simulink model "HANcoder_E407_TTA_Controller_v3"  (R2018b)
settings: Solver=FixedStepDiscrete  StartTime=0.0  StopTime=1  FixedStep=0.01  RelTol=1e-3
PreLoadFcn:
  | librarySetup
  | eval([bdroot,'_startup']) %Calling [modelName]_startup.m
values from neighbouring files (symbols this model uses):
  basic_cycle_duration_bc0 = TM_Reset_Board   + COMP_duration    (= 212)    [HANcoder_E407_TTA_Controller_v3_startup.m]
  basic_cycle_duration_bc1 = TM_Reset_Var_bc1 + COMP_duration    (= 288)    [HANcoder_E407_TTA_Controller_v3_startup.m]
  comm_delay_estimation1 = round(comm_delay_measured1*hardware_granularity/frequency_IRQ)    [HANcoder_E407_TTA_Controller_v3_startup.m]
  comm_delay_estimation2 = round(comm_delay_measured2*hardware_granularity/frequency_IRQ)    [HANcoder_E407_TTA_Controller_v3_startup.m]
  COMM_Period = 40    [HANcoder_E407_TTA_Controller_v3_startup.m]
  COMM_Phase1 = 5    [HANcoder_E407_TTA_Controller_v3_startup.m]
  COMM_Phase2 = 8    [HANcoder_E407_TTA_Controller_v3_startup.m]
  COMP_duration = 4    [HANcoder_E407_TTA_Controller_v3_startup.m]
  Controller1_Board = 1    [HANcoder_E407_TTA_Controller_v3_startup.m]
  Controller2_Board = 2    [HANcoder_E407_TTA_Controller_v3_startup.m]
  Controller3_Board = 3    [HANcoder_E407_TTA_Controller_v3_startup.m]
  delta_a_set = Simulink.Parameter    [HANcoder_E407_TTA_Controller_v3_startup.m]
  delta_f_set = Simulink.Parameter    [HANcoder_E407_TTA_Controller_v3_startup.m]
  delta_max = 1    [HANcoder_E407_TTA_Controller_v3_startup.m]
  delta_min = -1    [HANcoder_E407_TTA_Controller_v3_startup.m]
  delta_precision = 6    [HANcoder_E407_TTA_Controller_v3_startup.m]
  e_width = 0.1    [HANcoder_E407_TTA_Controller_v3_startup.m]
  frequency_IRQ = 100    [HANcoder_E407_TTA_Controller_v3_startup.m]
  HANtuneOverride = Simulink.Parameter    [HANcoder_E407_TTA_Controller_v3_startup.m]
  hardware_granularity = 1000000    [HANcoder_E407_TTA_Controller_v3_startup.m]
  I_a = 2.25    [HANcoder_E407_TTA_Controller_v3_startup.m]
  I_f = 2.25    [HANcoder_E407_TTA_Controller_v3_startup.m]
  idle_time_init = basic_cycle_duration_bc0 + basic_cycle_duration_bc1    (= 500)    [HANcoder_E407_TTA_Controller_v3_startup.m]
  Input_Gen_Board = 4    [HANcoder_E407_TTA_Controller_v3_startup.m]
  LA_Clock_Gr = 1    [HANcoder_E407_TTA_Controller_v3_startup.m]
  LA_COMM_Err = 0    [HANcoder_E407_TTA_Controller_v3_startup.m]
  LA_MEX_Flag = 0    [HANcoder_E407_TTA_Controller_v3_startup.m]
  LA_Task_Act = 1    [HANcoder_E407_TTA_Controller_v3_startup.m]
  m_v = 100.0    (= 100)    [HANcoder_E407_TTA_Controller_v3_startup.m]
  Master_Role = 1    [HANcoder_E407_TTA_Controller_v3_startup.m]
  matrix_cycle_duration = basic_cycle_duration_bc0 + basic_cycle_duration_bc1    (= 500)    [HANcoder_E407_TTA_Controller_v3_startup.m]
  matrix_rows = 2    [HANcoder_E407_TTA_Controller_v3_startup.m]
  max_num_msgs_CAN1 = 2^Tx_bit_number-1    (= 7)    [HANcoder_E407_TTA_Controller_v3_startup.m]
  max_num_msgs_CAN2 = max_num_msgs_CAN1    (= 7)    [HANcoder_E407_TTA_Controller_v3_startup.m]
  OutControl1_ID = 23    [HANcoder_E407_TTA_Controller_v3_startup.m]
  OutControl2_ID = 24    [HANcoder_E407_TTA_Controller_v3_startup.m]
  OutEmulator_ID = 25    [HANcoder_E407_TTA_Controller_v3_startup.m]
  R_al = 0.10    (= 0.1)    [HANcoder_E407_TTA_Controller_v3_startup.m]
  R_ar = 0.10    (= 0.1)    [HANcoder_E407_TTA_Controller_v3_startup.m]
  R_fl = 0.10    (= 0.1)    [HANcoder_E407_TTA_Controller_v3_startup.m]
  R_fr = 0.10    (= 0.1)    [HANcoder_E407_TTA_Controller_v3_startup.m]
  SensorValues_ID = 22    [HANcoder_E407_TTA_Controller_v3_startup.m]
  SetValues_ID = 21    [HANcoder_E407_TTA_Controller_v3_startup.m]
  Slave_Role = 2    [HANcoder_E407_TTA_Controller_v3_startup.m]
  speed_k_d = Simulink.Parameter    [HANcoder_E407_TTA_Controller_v3_startup.m]
  speed_k_i = Simulink.Parameter    [HANcoder_E407_TTA_Controller_v3_startup.m]
  speed_k_p = Simulink.Parameter    [HANcoder_E407_TTA_Controller_v3_startup.m]
  speed_max = 10    [HANcoder_E407_TTA_Controller_v3_startup.m]
  speed_min = -10    [HANcoder_E407_TTA_Controller_v3_startup.m]
  speed_precision = 3    [HANcoder_E407_TTA_Controller_v3_startup.m]
  Sync_ID = 1    [HANcoder_E407_TTA_Controller_v3_startup.m]
  tau_max = 5    [HANcoder_E407_TTA_Controller_v3_startup.m]
  tau_min = -5    [HANcoder_E407_TTA_Controller_v3_startup.m]
  tau_range = abs(tau_max) + abs(tau_min)    [HANcoder_E407_TTA_Controller_v3_startup.m]
  theta_max = 2    [HANcoder_E407_TTA_Controller_v3_startup.m]
  theta_min = -2    [HANcoder_E407_TTA_Controller_v3_startup.m]
  theta_precision = 5    [HANcoder_E407_TTA_Controller_v3_startup.m]
  Tl_a = 0.6    [HANcoder_E407_TTA_Controller_v3_startup.m]
  Tl_f = 0.6    [HANcoder_E407_TTA_Controller_v3_startup.m]
  TM_Check_Output_Control1 = TM_COMM_Output_Control1 + COMM_duration    (= 188)    [HANcoder_E407_TTA_Controller_v3_startup.m]
  TM_Check_Output_Control2 = TM_COMM_Output_Control2 + COMM_duration    (= 232)    [HANcoder_E407_TTA_Controller_v3_startup.m]
  TM_Check_Output_Emulator = TM_COMM_Output_Emulator + COMM_duration    (= 280)    [HANcoder_E407_TTA_Controller_v3_startup.m]
  TM_Check_Sensor_Values = TM_COMM_Sensor_Values + COMM_duration    (= 132)    [HANcoder_E407_TTA_Controller_v3_startup.m]
  TM_Check_Set_Values = TM_COMM_Set_Values + COMM_duration    (= 88)    [HANcoder_E407_TTA_Controller_v3_startup.m]
  TM_Check_Sync = TM_COMM_Sync   + COMM_duration    (= 40)    [HANcoder_E407_TTA_Controller_v3_startup.m]
  TM_Check_TOuts = TM_Count_Vote3 + COMP_duration    (= 196)    [HANcoder_E407_TTA_Controller_v3_startup.m]
  TM_Check_Vote1 = TM_COMM_Vote1  + COMM_duration    (= 92)    [HANcoder_E407_TTA_Controller_v3_startup.m]
  TM_Check_Vote2 = TM_COMM_Vote2  + COMM_duration    (= 140)    [HANcoder_E407_TTA_Controller_v3_startup.m]
  TM_Check_Vote3 = TM_COMM_Vote3  + COMM_duration    (= 188)    [HANcoder_E407_TTA_Controller_v3_startup.m]
  TM_COMM_Output_Control1 = TM_Velocity + COMP_duration    (= 148)    [HANcoder_E407_TTA_Controller_v3_startup.m]
  TM_COMM_Output_Control2 = TM_Check_Output_Control1 + COMP_duration    (= 192)    [HANcoder_E407_TTA_Controller_v3_startup.m]
  TM_COMM_Output_Emulator = TM_TMR + COMP_duration    (= 240)    [HANcoder_E407_TTA_Controller_v3_startup.m]
  TM_COMM_Sensor_Values = TM_Check_Set_Values + COMP_duration    (= 92)    [HANcoder_E407_TTA_Controller_v3_startup.m]
  TM_COMM_Set_Values = TM_Update_LT + COMP_duration    (= 48)    [HANcoder_E407_TTA_Controller_v3_startup.m]
  TM_COMM_Sync = basic_cycle_start    (= 0)    [HANcoder_E407_TTA_Controller_v3_startup.m]
  TM_COMM_Vote1 = TM_Vote_Dec    + COMP_duration    (= 52)    [HANcoder_E407_TTA_Controller_v3_startup.m]
  TM_COMM_Vote2 = TM_Count_Vote1 + COMP_duration    (= 100)    [HANcoder_E407_TTA_Controller_v3_startup.m]
  TM_COMM_Vote3 = TM_Count_Vote2 + COMP_duration    (= 148)    [HANcoder_E407_TTA_Controller_v3_startup.m]
  TM_Count_Vote1 = TM_Check_Vote1 + COMP_duration    (= 96)    [HANcoder_E407_TTA_Controller_v3_startup.m]
  TM_Count_Vote2 = TM_Check_Vote2 + COMP_duration    (= 144)    [HANcoder_E407_TTA_Controller_v3_startup.m]
  TM_Count_Vote3 = TM_Check_Vote3 + COMP_duration    (= 192)    [HANcoder_E407_TTA_Controller_v3_startup.m]
  TM_Data_bc0 = TM_COMM_Sync    (= 0)    [HANcoder_E407_TTA_Controller_v3_startup.m]
  TM_Data_bc1 = TM_Data_bc0(1:3)    [HANcoder_E407_TTA_Controller_v3_startup.m]
  TM_New_Master = TM_Check_TOuts + COMP_duration    (= 200)    [HANcoder_E407_TTA_Controller_v3_startup.m]
  TM_Reset_Board = TM_Reset_Var   + COMP_duration    (= 208)    [HANcoder_E407_TTA_Controller_v3_startup.m]
  TM_Reset_Var = TM_New_Master  + COMP_duration    (= 204)    [HANcoder_E407_TTA_Controller_v3_startup.m]
  TM_Reset_Var_bc1 = TM_Check_Output_Emulator + COMP_duration    (= 284)    [HANcoder_E407_TTA_Controller_v3_startup.m]
  TM_Steer = TM_Check_Sensor_Values + COMP_duration    (= 136)    [HANcoder_E407_TTA_Controller_v3_startup.m]
  TM_TMR = TM_Check_Output_Control2 + COMP_duration    (= 236)    [HANcoder_E407_TTA_Controller_v3_startup.m]
  TM_Torque = TM_Steer + COMP_duration    (= 140)    [HANcoder_E407_TTA_Controller_v3_startup.m]
  TM_Type_bc0 = COMM    (= 0)    [HANcoder_E407_TTA_Controller_v3_startup.m]
  TM_Type_bc1 = TM_Type_bc0(1:3)    [HANcoder_E407_TTA_Controller_v3_startup.m]
  TM_Update_LT = TM_Check_Sync  + COMP_duration    (= 44)    [HANcoder_E407_TTA_Controller_v3_startup.m]
  TM_Velocity = TM_Torque + COMP_duration    (= 144)    [HANcoder_E407_TTA_Controller_v3_startup.m]
  TM_Vote_Dec = TM_Update_LT   + COMP_duration    (= 48)    [HANcoder_E407_TTA_Controller_v3_startup.m]
  torque_a_k_d = Simulink.Parameter    [HANcoder_E407_TTA_Controller_v3_startup.m]
  torque_a_k_i = Simulink.Parameter    [HANcoder_E407_TTA_Controller_v3_startup.m]
  torque_a_k_p = Simulink.Parameter    [HANcoder_E407_TTA_Controller_v3_startup.m]
  torque_f_k_d = Simulink.Parameter    [HANcoder_E407_TTA_Controller_v3_startup.m]
  torque_f_k_i = Simulink.Parameter    [HANcoder_E407_TTA_Controller_v3_startup.m]
  torque_f_k_p = Simulink.Parameter    [HANcoder_E407_TTA_Controller_v3_startup.m]
  torque_precision = 4    [HANcoder_E407_TTA_Controller_v3_startup.m]
  v_set = Simulink.Parameter    [HANcoder_E407_TTA_Controller_v3_startup.m]
  Vehicle_Em_Board = 5    [HANcoder_E407_TTA_Controller_v3_startup.m]
  Vote1_ID = 11    [HANcoder_E407_TTA_Controller_v3_startup.m]
  Vote2_ID = 12    [HANcoder_E407_TTA_Controller_v3_startup.m]
  Vote3_ID = 13    [HANcoder_E407_TTA_Controller_v3_startup.m]
undefined symbols (not defined in the file or in its folder): A0, A1, A2, A3, A4, CON2
libraries: hdlsllib x352, HANcoder_STM32_Target x25, simulink x3, simulink_extras x1
(part 3 of 32)

== system HANcoder_E407_TTA_Controller_v3/HANcoder STM32 Target - E407-STM32 algorithm/Global Ticks Increment/CAN2 Recieve/RxID_CAN ==
  RxID : Inport
  Bus Creator4 : BusCreator  Inputs=8
  Bus Selector : BusSelector  OutputSignals=signal1,signal2,signal3,signal4,signal5,signal6,signal7,signal8,signal9
  Bus Creator{,1..3,5..9} (9 alike) : BusCreator  Inputs=9
  Constant : Constant  Value=Sync_ID
  Constant1 : Constant  Value=Vote1_ID
  Constant2 : Constant  Value=Vote2_ID
  Constant3 : Constant  Value=Vote3_ID
  Constant4 : Constant  Value=SetValues_ID
  Constant5 : Constant  Value=SensorValues_ID
  Constant6 : Constant  Value=OutControl1_ID
  Constant7 : Constant  Value=OutControl2_ID
  Constant8 : Constant  Value=OutEmulator_ID
  Equal{,1..8} (9 alike) : RelationalOperator  Operator===  OutDataTypeStr=boolean  RndMeth=Simplest
  OutControl1_ID_CAN : Subsystem
  OutControl2_ID_CAN : Subsystem
  OutEmulator_ID_CAN : Subsystem
  SensorValues_ID_CAN : Subsystem
  SetValues_ID_CAN : Subsystem
  Switch{,1..7} (8 alike) : Switch  Criteria=u2 > Threshold
  Sync_ID_CAN : Subsystem
  Vote1_ID_CAN : Subsystem
  Vote2_ID_CAN : Subsystem
  Vote3_ID_CAN : Subsystem
  CAN_new : Outport
  message : Outport  Port=2
  wires:
  Constant/1 -> Equal/2
  Equal/1 -> Sync_ID_CAN/Enable, Switch/2
  Constant1/1 -> Equal1/2
  Constant2/1 -> Equal2/2
  Constant3/1 -> Equal3/2
  Equal1/1 -> Vote1_ID_CAN/Enable, Switch1/2
  Equal2/1 -> Vote2_ID_CAN/Enable, Switch2/2
  Equal3/1 -> Vote3_ID_CAN/Enable, Switch3/2
  Sync_ID_CAN/1(CAN_new) -> Bus Creator/1
  Sync_ID_CAN/2(Out2) -> Bus Creator/2
  Sync_ID_CAN/3(Out3) -> Bus Creator/3
  Sync_ID_CAN/4(Out4) -> Bus Creator/4
  Sync_ID_CAN/5(Out5) -> Bus Creator/5
  Sync_ID_CAN/6(Out6) -> Bus Creator/6
  Sync_ID_CAN/7(Out7) -> Bus Creator/7
  Sync_ID_CAN/8(Out8) -> Bus Creator/8
  Sync_ID_CAN/9(Out9) -> Bus Creator/9
  Bus Creator/1 -> Switch/1
  Vote1_ID_CAN/1(CAN_new) -> Bus Creator1/1
  Vote1_ID_CAN/2(Out2) -> Bus Creator1/2
  Vote1_ID_CAN/3(Out3) -> Bus Creator1/3
  Vote1_ID_CAN/4(Out4) -> Bus Creator1/4
  Vote1_ID_CAN/5(Out5) -> Bus Creator1/5
  Vote1_ID_CAN/6(Out6) -> Bus Creator1/6
  Vote1_ID_CAN/7(Out7) -> Bus Creator1/7
  Vote1_ID_CAN/8(Out8) -> Bus Creator1/8
  Vote1_ID_CAN/9(Out9) -> Bus Creator1/9
  Bus Creator1/1 -> Switch1/1
  Vote2_ID_CAN/1(CAN_new) -> Bus Creator2/1
  Vote2_ID_CAN/2(Out2) -> Bus Creator2/2
  Vote2_ID_CAN/3(Out3) -> Bus Creator2/3
  Vote2_ID_CAN/4(Out4) -> Bus Creator2/4
  Vote2_ID_CAN/6(Out6) -> Bus Creator2/6
  Vote2_ID_CAN/5(Out5) -> Bus Creator2/5
  Vote2_ID_CAN/7(Out7) -> Bus Creator2/7
  Vote2_ID_CAN/8(Out8) -> Bus Creator2/8
  Vote2_ID_CAN/9(Out9) -> Bus Creator2/9
  Bus Creator2/1 -> Switch2/1
  Vote3_ID_CAN/1(CAN_new) -> Bus Creator3/1
  Vote3_ID_CAN/2(Out2) -> Bus Creator3/2
  Vote3_ID_CAN/3(Out3) -> Bus Creator3/3
  Vote3_ID_CAN/4(Out4) -> Bus Creator3/4
  Vote3_ID_CAN/5(Out5) -> Bus Creator3/5
  Vote3_ID_CAN/6(Out6) -> Bus Creator3/6
  Vote3_ID_CAN/7(Out7) -> Bus Creator3/7
  Vote3_ID_CAN/8(Out8) -> Bus Creator3/8
  Vote3_ID_CAN/9(Out9) -> Bus Creator3/9
  Bus Creator3/1 -> Switch3/1
  Switch1/1 -> Switch/3
  Switch2/1 -> Switch1/3
  Switch/1 -> Bus Selector/1
  Bus Selector/1 -> CAN_new/1  "<signal1>"
  Bus Creator4/1 -> message/1
  Bus Selector/2 -> Bus Creator4/1  "<signal2>"
  Bus Selector/6 -> Bus Creator4/5  "<signal6>"
  Bus Selector/7 -> Bus Creator4/6  "<signal7>"
  Bus Selector/8 -> Bus Creator4/7  "<signal8>"
  Bus Selector/9 -> Bus Creator4/8  "<signal9>"
  Bus Selector/3 -> Bus Creator4/2  "<signal3>"
  Bus Selector/4 -> Bus Creator4/3  "<signal4>"
  Bus Selector/5 -> Bus Creator4/4  "<signal5>"
  Switch3/1 -> Switch2/3
  Switch4/1 -> Switch3/3
  Switch5/1 -> Switch4/3
  SetValues_ID_CAN/9(Out9) -> Bus Creator5/9
  SetValues_ID_CAN/8(Out8) -> Bus Creator5/8
  SetValues_ID_CAN/7(Out7) -> Bus Creator5/7
  SetValues_ID_CAN/6(Out6) -> Bus Creator5/6
  SetValues_ID_CAN/5(Out5) -> Bus Creator5/5
  SetValues_ID_CAN/2(Out2) -> Bus Creator5/2
  SetValues_ID_CAN/1(CAN_new) -> Bus Creator5/1
  SetValues_ID_CAN/3(Out3) -> Bus Creator5/3
  SetValues_ID_CAN/4(Out4) -> Bus Creator5/4
  Bus Creator5/1 -> Switch4/1
  Constant4/1 -> Equal4/2
  Equal4/1 -> SetValues_ID_CAN/Enable, Switch4/2
  Equal5/1 -> Switch5/2, SensorValues_ID_CAN/Enable
  Constant5/1 -> Equal5/2
  Bus Creator6/1 -> Switch5/1
  SensorValues_ID_CAN/4(Out4) -> Bus Creator6/4
  SensorValues_ID_CAN/3(Out3) -> Bus Creator6/3
  SensorValues_ID_CAN/1(CAN_new) -> Bus Creator6/1
  SensorValues_ID_CAN/2(Out2) -> Bus Creator6/2
  SensorValues_ID_CAN/5(Out5) -> Bus Creator6/5
  SensorValues_ID_CAN/6(Out6) -> Bus Creator6/6
  SensorValues_ID_CAN/7(Out7) -> Bus Creator6/7
  SensorValues_ID_CAN/8(Out8) -> Bus Creator6/8
  SensorValues_ID_CAN/9(Out9) -> Bus Creator6/9
  OutControl1_ID_CAN/9(Out9) -> Bus Creator7/9
  OutControl1_ID_CAN/8(Out8) -> Bus Creator7/8
  OutControl1_ID_CAN/7(Out7) -> Bus Creator7/7
  OutControl1_ID_CAN/6(Out6) -> Bus Creator7/6
  OutControl1_ID_CAN/5(Out5) -> Bus Creator7/5
  OutControl1_ID_CAN/2(Out2) -> Bus Creator7/2
  OutControl1_ID_CAN/1(CAN_new) -> Bus Creator7/1
  OutControl1_ID_CAN/3(Out3) -> Bus Creator7/3
  OutControl1_ID_CAN/4(Out4) -> Bus Creator7/4
  Constant6/1 -> Equal6/2
  Equal6/1 -> Switch6/2, OutControl1_ID_CAN/Enable
  Bus Creator7/1 -> Switch6/1
  Bus Creator8/1 -> Switch7/1
  Equal7/1 -> Switch7/2, OutControl2_ID_CAN/Enable
  Constant7/1 -> Equal7/2
  OutControl2_ID_CAN/4(Out4) -> Bus Creator8/4
  OutControl2_ID_CAN/3(Out3) -> Bus Creator8/3
  OutControl2_ID_CAN/1(CAN_new) -> Bus Creator8/1
  OutControl2_ID_CAN/2(Out2) -> Bus Creator8/2
  OutControl2_ID_CAN/5(Out5) -> Bus Creator8/5
  OutControl2_ID_CAN/6(Out6) -> Bus Creator8/6
  OutControl2_ID_CAN/7(Out7) -> Bus Creator8/7
  OutControl2_ID_CAN/8(Out8) -> Bus Creator8/8
  OutControl2_ID_CAN/9(Out9) -> Bus Creator8/9
  OutEmulator_ID_CAN/9(Out9) -> Bus Creator9/9
  OutEmulator_ID_CAN/8(Out8) -> Bus Creator9/8
  OutEmulator_ID_CAN/7(Out7) -> Bus Creator9/7
  OutEmulator_ID_CAN/6(Out6) -> Bus Creator9/6
  OutEmulator_ID_CAN/5(Out5) -> Bus Creator9/5
  OutEmulator_ID_CAN/2(Out2) -> Bus Creator9/2
  OutEmulator_ID_CAN/1(CAN_new) -> Bus Creator9/1
  OutEmulator_ID_CAN/3(Out3) -> Bus Creator9/3
  OutEmulator_ID_CAN/4(Out4) -> Bus Creator9/4
  Constant8/1 -> Equal8/2
  RxID/1 -> Equal2/1, Equal6/1, Equal7/1, Equal8/1, Equal5/1, Equal4/1, Equal3/1, Equal1/1, Equal/1
  Equal8/1 -> OutEmulator_ID_CAN/Enable
  Bus Creator9/1 -> Switch7/3
  Switch7/1 -> Switch6/3
  Switch6/1 -> Switch5/3

== system HANcoder_E407_TTA_Controller_v3/HANcoder STM32 Target - E407-STM32 algorithm/Global Ticks Increment/CAN2 Recieve/Update message buffers ==
  note: Logic Analyzer - DEBUG
      | Message received!
  note: CAN_Rx stop listening
  note: Received message
      | ready for processing
  note: Local time when the
      | message is received
  message : Inport  OutDataTypeStr=Bus: msg_buffer_type
  Enable : EnablePort
  Bus Selector : BusSelector  OutputSignals=signal2,signal3,signal4,signal5,signal6,signal7,signal8,signal9
  Cast To Double : DataTypeConversion  OutDataTypeStr=double
  Data Store Write : DataStoreWrite  DataStoreName=Toggle_Pin_A0
  Data Store Write1 : DataStoreWrite  DataStoreName=Msg_Rx_CAN2  DataStoreElements=Msg_Rx_CAN2.Buffer_1#Msg_Rx_CAN2.Buffer_2#Msg_Rx_CAN2.Buffer_3#Msg_Rx_CAN2.Buffer_4#Msg_Rx_CAN2.Buffer_5#Msg_Rx_CAN2.Buffer_6#Msg_Rx_CAN2.Buffer_7#Msg_Rx_CAN2.Buffer_8
  Data Store Write2 : DataStoreWrite  DataStoreName=New_Msg_Ready_CAN2
  Data Store Write5 : DataStoreWrite  DataStoreName=Rx_State_CAN2
  Data Store Write6 : DataStoreWrite  DataStoreName=Msg_Rx_Ticks_CAN2
  Idle_State : Constant  Value=3  OutDataTypeStr=uint8
  Local_Time : DataStoreRead  DataStoreName=Local_Ticks
  SET : Constant  OutDataTypeStr=boolean
  Terminator : Terminator
  wires:
  Local_Time/1 -> Data Store Write6/1  "Rx_msg_ticks_CAN2"
  SET/1 -> Data Store Write2/1, Data Store Write/1
  message/1 -> Bus Selector/1
  Idle_State/1 -> Data Store Write5/1
  Bus Selector/1 -> Cast To Double/1, Data Store Write1/1  "<signal2>"
  Bus Selector/2 -> Data Store Write1/2  "<signal3>"
  Bus Selector/3 -> Data Store Write1/3  "<signal4>"
  Bus Selector/4 -> Data Store Write1/4  "<signal5>"
  Bus Selector/5 -> Data Store Write1/5  "<signal6>"
  Bus Selector/6 -> Data Store Write1/6  "<signal7>"
  Bus Selector/7 -> Data Store Write1/7  "<signal8>"
  Bus Selector/8 -> Data Store Write1/8  "<signal9>"
  Cast To Double/1 -> Terminator/1  "Rx_temporal_msg_CAN2"

== system HANcoder_E407_TTA_Controller_v3/HANcoder STM32 Target - E407-STM32 algorithm/Global Ticks Increment/CAN2 Send/CAN send1 ==
  In1 : Inport
  In2 : Inport  Port=2
  In3 : Inport  Port=3
  In4 : Inport  Port=4
  In5 : Inport  Port=5
  In6 : Inport  Port=6
  In7 : Inport  Port=7
  In8 : Inport  Port=8
  In9 : Inport  Port=9
  S-Function : M-S-Function  FunctionName=sfcn_can_send  Parameters=tsamp, canBus, frameType, inputNumber, dataType, byteOrder
  wires:
  In1/1 -> S-Function/1
  In2/1 -> S-Function/2
  In3/1 -> S-Function/3
  In4/1 -> S-Function/4
  In5/1 -> S-Function/5
  In6/1 -> S-Function/6
  In7/1 -> S-Function/7
  In8/1 -> S-Function/8
  In9/1 -> S-Function/9

== system HANcoder_E407_TTA_Controller_v3/HANcoder STM32 Target - E407-STM32 algorithm/Global Ticks Increment/Measure EXecution time/DEBUG - Toggle digital pin A3 ==
  note: Change pin state
  note: Toggle pin data stored
  Enable : EnablePort
  Constant : Constant  OutDataTypeStr=boolean
  Constant1 : Constant  Value=0  OutDataTypeStr=boolean
  Data Store Read : DataStoreRead  DataStoreName=A3_Pin_State
  Data Store Read1 : DataStoreRead  DataStoreName=A3_Pin_State
  Data Store Write1 : DataStoreWrite  DataStoreName=A3_Pin_State
  Digital Output1 : HANcoder_STM32_Target/STM32-E407/Digital Outputs/Digital Output  Tag=HANcoder_TARGET_STM32_E407  pinID=CON2 - A3  config=Open drain  tsamp=-1
      settings: SourceProductName=HANcoder STM32 Target
  Switch : Switch  Criteria=u2 > Threshold
  wires:
  Switch/1 -> Data Store Write1/1
  Data Store Read/1 -> Switch/2
  Constant/1 -> Switch/3
  Constant1/1 -> Switch/1
  Data Store Read1/1 -> Digital Output1/1

== system HANcoder_E407_TTA_Controller_v3/HANcoder STM32 Target - E407-STM32 algorithm/Global Ticks Increment/CAN Management/Initialization/Delay ==
  note: Update counter
      | < +1 tick every activation >
  note: Reset local counter
      | < for next activation >
  note: End of Delay
  Input : Inport
  Add2 : Sum
  Data Store Read : DataStoreRead  DataStoreName=Delay_Counter
  Data Store Read1 : DataStoreRead  DataStoreName=Delay_Counter
  Data Store Write2 : DataStoreWrite  DataStoreName=Delay_Counter
  GreaterThan : RelationalOperator  OutDataTypeStr=boolean  RndMeth=Simplest
  Increment1 : Constant  OutDataTypeStr=double
  Reset : Constant  Value=-1  OutDataTypeStr=double
  Switch : Switch  Criteria=u2 > Threshold
  Output : Outport
  wires:
  Data Store Read/1 -> Add2/1
  Increment1/1 -> Add2/2
  Data Store Read1/1 -> GreaterThan/1
  Input/1 -> GreaterThan/2
  GreaterThan/1 -> Switch/2, Output/1
  Add2/1 -> Switch/3
  Reset/1 -> Switch/1
  Switch/1 -> Data Store Write2/1

== system HANcoder_E407_TTA_Controller_v3/HANcoder STM32 Target - E407-STM32 algorithm/Global Ticks Increment/CAN Management/Initialization/RoleID and Global Time init ==
  note: Sync msg received!
  note: Reset variables
  note: Finish Initialization
  note: Role_ID Initialization
  Timeout Initialization : Inport
  Reference message received : Inport  Port=2
  Enable : EnablePort
  Constant : Constant  Priority=4  Value=Master_Role
  Constant1 : Constant  Priority=3  Value=Slave_Role
  Data Store Read : DataStoreRead  Priority=5  DataStoreName=Role_ID
  Data Store Write : DataStoreWrite  Priority=8  DataStoreName=Role_ID
  Data Store Write2 : DataStoreWrite  Priority=18  DataStoreName=Delay_Counter
  Data Store Write3 : DataStoreWrite  Priority=12  DataStoreName=New_Msg_Ready_CAN1
  Data Store Write4 : DataStoreWrite  Priority=16  DataStoreName=Initialization_Timeout
  Data Store Write5 : DataStoreWrite  Priority=14  DataStoreName=New_Msg_Ready_CAN2
  Global Time Initialization Master : Subsystem  Priority=2
  Global Time Initialization Slave : Subsystem  Priority=1
  RESET : Constant  Priority=15  Value=0  OutDataTypeStr=boolean
  RESET1 : Constant  Priority=17  Value=0  OutDataTypeStr=double
  RESET2 : Constant  Priority=11  Value=0  OutDataTypeStr=boolean
  RESET3 : Constant  Priority=13  Value=0  OutDataTypeStr=boolean
  SET : Constant  Priority=19
  Switch1 : Switch  Priority=6  Criteria=u2 > Threshold
  Switch2 : Switch  Priority=7  Criteria=u2 > Threshold
  Finish Initialization : Outport  OutputWhenDisabled=reset  InitialOutput=0
  wires:
  Switch1/1 -> Switch2/3
  Reference message received/1 -> Global Time Initialization Slave/Enable, Switch2/2
  Data Store Read/1 -> Switch1/3
  SET/1 -> Finish Initialization/1
  Constant/1 -> Switch1/1
  Constant1/1 -> Switch2/1
  Switch2/1 -> Data Store Write/1
  RESET/1 -> Data Store Write4/1
  Timeout Initialization/1 -> Switch1/2, Global Time Initialization Master/Enable
  RESET1/1 -> Data Store Write2/1
  RESET2/1 -> Data Store Write3/1
  RESET3/1 -> Data Store Write5/1

== system HANcoder_E407_TTA_Controller_v3/HANcoder STM32 Target - E407-STM32 algorithm/Global Ticks Increment/CAN Management/LT_Update Desync_Positive/Local Time Update with Positive Desync ==
  note: Positive Desync with respect to the master
      | If the desync is positive, we have to update the
      | Local Time to be "in the future". This is problematic
      | because we do not want the schedule to go ahead
      | of time and forget to do any task. That is why we
      | correct the desync in small steps.
  note: End condition
  note: Desync counter
      | reduction
  note: Local Time Update
  note: Current Local Time correction
  Ticks until next COMP : Inport
  Cast : DataTypeConversion  Priority=13  OutDataTypeStr=uint16
  Constant : Constant  Value=0
  Data Store Read : DataStoreRead  DataStoreName=Local_Ticks
  Data Store Read2 : DataStoreRead  DataStoreName=Desync_Ticks
  Data Store Write : DataStoreWrite  DataStoreName=Desync_Positive
  Data Store Write1 : DataStoreWrite  Priority=14  DataStoreName=Local_Ticks  DataStoreElements=Local_Ticks
  Data Store Write2 : DataStoreWrite  DataStoreName=Desync_Ticks
  Equal : RelationalOperator  Operator=<=  OutDataTypeStr=boolean  RndMeth=Simplest
  GreaterThan : RelationalOperator  Operator=<=  OutDataTypeStr=boolean  RndMeth=Simplest
  Minus : Sum  Priority=12
  Minus1 : Sum  Inputs=+-
  NOT : Logic  Operator=NOT  IconShape=distinctive  AllPortsSameDT=off  OutDataTypeStr=boolean
  Switch : Switch  Criteria=u2 > Threshold
  wires:
  Ticks until next COMP/1 -> Switch/1, GreaterThan/1
  Data Store Read/1 -> Minus/1
  Cast/1 -> Data Store Write1/1
  Minus/1 -> Cast/1
  Data Store Read2/1 -> Switch/3, GreaterThan/2, Minus1/2
  Minus1/1 -> Equal/1, Data Store Write2/1
  Constant/1 -> Equal/2
  Equal/1 -> NOT/1
  NOT/1 -> Data Store Write/1
  GreaterThan/1 -> Switch/2
  Switch/1 -> Minus1/1, Minus/2

== system HANcoder_E407_TTA_Controller_v3/HANcoder STM32 Target - E407-STM32 algorithm/Global Ticks Increment/CAN Management/Matrix Cycle Manager/Controller Matrix Cycle ==
  note: Nodes Voting
      | Own_Vote:
      |    Individual vote of current node
      |
      |
      | Votes_count:
      |    Count of all received votes
  basic_cycle : Inport
  Enable : EnablePort  PropagateVarSize=During execution
  Bus Selector : BusSelector  OutputSignals=signal1,signal2,signal3,signal4
  Bus Creator : BusCreator  Inputs=4
  Bus Creator1 : BusCreator  Inputs=4
  Constant : Constant  Value=0
  Constant1 : Constant
  Data Store Memory : DataStoreMemory  DataStoreName=msg_count_DEBUG  ReadBeforeWriteMsg=warning  WriteAfterWriteMsg=warning  WriteAfterReadMsg=warning  ShowAdditionalParam=off
  Data Store Memory1 : DataStoreMemory  DataStoreName=Board1_error_counter  ReadBeforeWriteMsg=warning  WriteAfterWriteMsg=warning  WriteAfterReadMsg=warning  ShowAdditionalParam=off  OutMin=0  OutMax=4294967294  OutDataTypeStr=double
  Data Store Memory12 : DataStoreMemory  Priority=30  DataStoreName=Own_Vote  ReadBeforeWriteMsg=warning  WriteAfterWriteMsg=warning  WriteAfterReadMsg=warning  ShowAdditionalParam=off  OutDataTypeStr=uint8
  Data Store Memory2 : DataStoreMemory  DataStoreName=Board2_error_counter  ReadBeforeWriteMsg=warning  WriteAfterWriteMsg=warning  WriteAfterReadMsg=warning  ShowAdditionalParam=off  OutMin=0  OutMax=4294967294  OutDataTypeStr=double
  Data Store Memory3 : DataStoreMemory  DataStoreName=Board3_error_counter  ReadBeforeWriteMsg=warning  WriteAfterWriteMsg=warning  WriteAfterReadMsg=warning  ShowAdditionalParam=off  OutMin=0  OutMax=4294967294  OutDataTypeStr=double
  Data Store Memory4 : DataStoreMemory  Priority=30  DataStoreName=BC0_Vote2_processed  ReadBeforeWriteMsg=warning  WriteAfterWriteMsg=warning  WriteAfterReadMsg=warning  ShowAdditionalParam=off  OutDataTypeStr=boolean
  Data Store Memory5 : DataStoreMemory  Priority=30  DataStoreName=BC0_Vote3_processed  ReadBeforeWriteMsg=warning  WriteAfterWriteMsg=warning  WriteAfterReadMsg=warning  ShowAdditionalParam=off  OutDataTypeStr=boolean
  Data Store Memory6 : DataStoreMemory  Priority=30  DataStoreName=BC0_Vote1_processed  ReadBeforeWriteMsg=warning  WriteAfterWriteMsg=warning  WriteAfterReadMsg=warning  ShowAdditionalParam=off  OutDataTypeStr=boolean
  Data Store Memory9 : DataStoreMemory  Priority=30  DataStoreName=Votes_count  ReadBeforeWriteMsg=warning  WriteAfterWriteMsg=warning  WriteAfterReadMsg=warning  ShowAdditionalParam=off  OutDataTypeStr=Bus: vote_array
  Equal : RelationalOperator  Operator===  OutDataTypeStr=boolean  RndMeth=Simplest
  Equal1 : RelationalOperator  Operator===  OutDataTypeStr=boolean  RndMeth=Simplest
  Matrix_Cycle_Observation_DEBUG : Subsystem
  Switch : Switch  Criteria=u2 > Threshold
  controller basic cycle 0 : Subsystem
  controller basic cycle 1 : Subsystem
  msg_count_DEBUG observer : Subsystem
  Send_CAN1 : Outport  OutputWhenDisabled=reset  InitialOutput=0
  Send_CAN2 : Outport  Port=2  OutputWhenDisabled=reset  InitialOutput=0
  Receive_CAN1 : Outport  Port=3  OutputWhenDisabled=reset  InitialOutput=0
  Receive_CAN2 : Outport  Port=4  OutputWhenDisabled=reset  InitialOutput=0
  wires:
  Bus Creator1/1 -> Switch/3
  Bus Selector/1 -> Send_CAN1/1  "<signal1>"
  Constant/1 -> Equal/2
  controller basic cycle 0/4(Receive_Message_CAN2) -> Bus Creator/4
  Equal/1 -> Switch/2, controller basic cycle 0/Enable
  basic_cycle/1 -> Equal1/1, Equal/1
  controller basic cycle 0/2(Send_Message_CAN2) -> Bus Creator/2
  Equal1/1 -> controller basic cycle 1/Enable
  Bus Selector/2 -> Send_CAN2/1  "<signal2>"
  Constant1/1 -> Equal1/2
  Bus Selector/4 -> Receive_CAN2/1  "<signal4>"
  controller basic cycle 0/3(Receive_Message_CAN1) -> Bus Creator/3
  controller basic cycle 0/1(Send_Message_CAN1) -> Bus Creator/1
  Bus Creator/1 -> Switch/1
  controller basic cycle 1/4(Receive_Message_CAN2) -> Bus Creator1/4
  Switch/1 -> Bus Selector/1
  controller basic cycle 1/3(Receive_Message_CAN1) -> Bus Creator1/3
  Bus Selector/3 -> Receive_CAN1/1  "<signal3>"
  controller basic cycle 1/2(Send_Message_CAN2) -> Bus Creator1/2
  controller basic cycle 1/1(Send_Message_CAN1) -> Bus Creator1/1

== system HANcoder_E407_TTA_Controller_v3/HANcoder STM32 Target - E407-STM32 algorithm/Global Ticks Increment/CAN Management/Matrix Cycle Manager/Input Generator Matrix Cycle ==
  basic_cycle : Inport
  Enable : EnablePort  PropagateVarSize=During execution
  Bus Selector : BusSelector  OutputSignals=signal1,signal2,signal3,signal4
  Bus Creator : BusCreator  Inputs=4
  Bus Creator1 : BusCreator  Inputs=4
  Constant : Constant  Value=0
  Constant1 : Constant
  Data Store Memory : DataStoreMemory  DataStoreName=msg_count_DEBUG  ReadBeforeWriteMsg=warning  WriteAfterWriteMsg=warning  WriteAfterReadMsg=warning  ShowAdditionalParam=off
  Equal : RelationalOperator  Operator===  OutDataTypeStr=boolean  RndMeth=Simplest
  Equal1 : RelationalOperator  Operator===  OutDataTypeStr=boolean  RndMeth=Simplest
  Matrix_Cycle_Observation_DEBUG : Subsystem
  Switch : Switch  Criteria=u2 > Threshold
  input generator basic cycle 0 : Subsystem
  input generator basic cycle 1 : Subsystem
  msg_count_DEBUG observer : Subsystem
  Send_CAN1 : Outport  OutputWhenDisabled=reset  InitialOutput=0
  Send_CAN2 : Outport  Port=2  OutputWhenDisabled=reset  InitialOutput=0
  Receive_CAN1 : Outport  Port=3  OutputWhenDisabled=reset  InitialOutput=0
  Receive_CAN2 : Outport  Port=4  OutputWhenDisabled=reset  InitialOutput=0
  wires:
  input generator basic cycle 1/1(Send_Message_CAN1) -> Bus Creator1/1
  input generator basic cycle 1/2(Send_Message_CAN2) -> Bus Creator1/2
  Bus Selector/3 -> Receive_CAN1/1  "<signal3>"
  input generator basic cycle 1/3(Receive_Message_CAN1) -> Bus Creator1/3
  Switch/1 -> Bus Selector/1
  input generator basic cycle 1/4(Receive_Message_CAN2) -> Bus Creator1/4
  Bus Creator/1 -> Switch/1
  input generator basic cycle 0/1(Send_Message_CAN1) -> Bus Creator/1
  input generator basic cycle 0/3(Receive_Message_CAN1) -> Bus Creator/3
  Bus Selector/4 -> Receive_CAN2/1  "<signal4>"
  Constant1/1 -> Equal1/2
  Bus Selector/2 -> Send_CAN2/1  "<signal2>"
  Equal1/1 -> input generator basic cycle 1/Enable
  input generator basic cycle 0/2(Send_Message_CAN2) -> Bus Creator/2
  basic_cycle/1 -> Equal/1, Equal1/1
  Equal/1 -> input generator basic cycle 0/Enable, Switch/2
  input generator basic cycle 0/4(Receive_Message_CAN2) -> Bus Creator/4
  Constant/1 -> Equal/2
  Bus Selector/1 -> Send_CAN1/1  "<signal1>"
  Bus Creator1/1 -> Switch/3

== system HANcoder_E407_TTA_Controller_v3/HANcoder STM32 Target - E407-STM32 algorithm/Global Ticks Increment/CAN Management/Matrix Cycle Manager/Vehicle Emulator Matrix Cycle ==
  note: Flag for missing controller torques
      | output. If this is set, no calculations
      | are done.
  note: This is evaluated during OutputCOMM
      | task in bc1
  note: Time from last time we got
      | data from the controller
  note: Torque values from controller
      |    <CONTROLLER OUTPUT>
  note: These values are calculated during bc0 with Controller's
      | torque values, and sent back to the controller in bc1
  note: Wheel displacement estimation
      |         <SENSOR VALUES>
  note: These other values are received at the end of bc1 from
      | the Controller and used during bc0 to calculate the thetas
  basic_cycle : Inport
  Enable : EnablePort  PropagateVarSize=During execution
  Bus Selector : BusSelector  OutputSignals=signal1,signal2,signal3,signal4
  Bus Creator : BusCreator  Inputs=4
  Bus Creator1 : BusCreator  Inputs=4
  Constant : Constant  Value=0
  Constant1 : Constant
  Data Store Memory : DataStoreMemory  DataStoreName=msg_count_DEBUG  ReadBeforeWriteMsg=warning  WriteAfterWriteMsg=warning  WriteAfterReadMsg=warning  ShowAdditionalParam=off
  Data Store Memory1 : DataStoreMemory  DataStoreName=torque_fr  ReadBeforeWriteMsg=warning  WriteAfterWriteMsg=warning  WriteAfterReadMsg=warning  ShowAdditionalParam=off
  Data Store Memory2 : DataStoreMemory  DataStoreName=torque_ar  ReadBeforeWriteMsg=warning  WriteAfterWriteMsg=warning  WriteAfterReadMsg=warning  ShowAdditionalParam=off
  Data Store Memory3 : DataStoreMemory  DataStoreName=torque_fl  ReadBeforeWriteMsg=warning  WriteAfterWriteMsg=warning  WriteAfterReadMsg=warning  ShowAdditionalParam=off
  Data Store Memory4 : DataStoreMemory  DataStoreName=torque_al  ReadBeforeWriteMsg=warning  WriteAfterWriteMsg=warning  WriteAfterReadMsg=warning  ShowAdditionalParam=off
  Data Store Memory5 : DataStoreMemory  DataStoreName=rx_data_incr_time  ReadBeforeWriteMsg=warning  WriteAfterWriteMsg=warning  WriteAfterReadMsg=warning  ShowAdditionalParam=off
  Data Store Memory6 : DataStoreMemory  DataStoreName=controller_msg_missed  ReadBeforeWriteMsg=warning  WriteAfterWriteMsg=warning  WriteAfterReadMsg=warning  ShowAdditionalParam=off
  Data Store Memory60 : DataStoreMemory  DataStoreName=theta_fr_incr  ReadBeforeWriteMsg=warning  WriteAfterWriteMsg=warning  WriteAfterReadMsg=warning  ShowAdditionalParam=off
  Data Store Memory61 : DataStoreMemory  DataStoreName=theta_fl_incr  ReadBeforeWriteMsg=warning  WriteAfterWriteMsg=warning  WriteAfterReadMsg=warning  ShowAdditionalParam=off
  Data Store Memory73 : DataStoreMemory  DataStoreName=theta_ar_incr  ReadBeforeWriteMsg=warning  WriteAfterWriteMsg=warning  WriteAfterReadMsg=warning  ShowAdditionalParam=off
  Data Store Memory74 : DataStoreMemory  DataStoreName=theta_al_incr  ReadBeforeWriteMsg=warning  WriteAfterWriteMsg=warning  WriteAfterReadMsg=warning  ShowAdditionalParam=off
  Equal : RelationalOperator  Operator===  OutDataTypeStr=boolean  RndMeth=Simplest
  Equal1 : RelationalOperator  Operator===  OutDataTypeStr=boolean  RndMeth=Simplest
  Matrix_Cycle_Observation_DEBUG : Subsystem
  Switch : Switch  Criteria=u2 > Threshold
  msg_count_DEBUG observer : Subsystem
  vehicle emulator basic cycle 0 : Subsystem
  vehicle emulator basic cycle 1 : Subsystem
  Send_CAN1 : Outport  OutputWhenDisabled=reset  InitialOutput=0
  Send_CAN2 : Outport  Port=2  OutputWhenDisabled=reset  InitialOutput=0
  Receive_CAN1 : Outport  Port=3  OutputWhenDisabled=reset  InitialOutput=0
  Receive_CAN2 : Outport  Port=4  OutputWhenDisabled=reset  InitialOutput=0
  wires:
  Bus Creator1/1 -> Switch/3
  Bus Selector/1 -> Send_CAN1/1  "<signal1>"
  Constant/1 -> Equal/2
  vehicle emulator basic cycle 0/4(Receive_Message_CAN2) -> Bus Creator/4
  Equal/1 -> Switch/2, vehicle emulator basic cycle 0/Enable
  basic_cycle/1 -> Equal1/1, Equal/1
  vehicle emulator basic cycle 0/2(Send_Message_CAN2) -> Bus Creator/2
  Equal1/1 -> vehicle emulator basic cycle 1/Enable
  Bus Selector/2 -> Send_CAN2/1  "<signal2>"
  Constant1/1 -> Equal1/2
  Bus Selector/4 -> Receive_CAN2/1  "<signal4>"
  vehicle emulator basic cycle 0/3(Receive_Message_CAN1) -> Bus Creator/3
  vehicle emulator basic cycle 0/1(Send_Message_CAN1) -> Bus Creator/1
  Bus Creator/1 -> Switch/1
  vehicle emulator basic cycle 1/4(Receive_Message_CAN2) -> Bus Creator1/4
  Switch/1 -> Bus Selector/1
  vehicle emulator basic cycle 1/3(Receive_Message_CAN1) -> Bus Creator1/3
  Bus Selector/3 -> Receive_CAN1/1  "<signal3>"
  vehicle emulator basic cycle 1/2(Send_Message_CAN2) -> Bus Creator1/2
  vehicle emulator basic cycle 1/1(Send_Message_CAN1) -> Bus Creator1/1

== system HANcoder_E407_TTA_Controller_v3/HANcoder STM32 Target - E407-STM32 algorithm/Global Ticks Increment/CAN1 Recieve/RxID_CAN/OutControl1_ID_CAN ==
  Enable : EnablePort
  CAN receive1 : Subsystem  Tag=HANcoder_TARGET_STM32_E407  AncestorBlock=HANcoder_STM32_Target/STM32-E407/CAN/CAN/CAN receive  mask(CAN receive){canBus=CAN 1, outputNumber=8, dataType=uint8, byteOrder=off, tsamp=-1}
      mask prompts: canBus "CAN channel"; outputNumber "Output ports"; dataType "Output datatype"; byteOrder "Byte order: Checked = MSB first, unchecked = LSB first."; tsamp "Sample time"
      mask help:
      | Function
      | ==========
      | Receive the newest message from the specified CAN channel.
      |
      | Parameters
      | ==========
      | CAN channel:             The CAN channel to send the message on.
      | Output ports:             The amount of output ports
      | Output datatype:       The datatype of the output ports
      | Byte order:                 Select MSB or LSB first
      | Sample time:              -1 or divisible by base sample time [seconds]
      |
      | Input
      | ==========
      | Port 1:                       CAN ID(uint32) in hexadecimal ie: hex2dec('0a')
      |
      | Output
      | ==========
      | Port 1:                       Checks for new message(int8)
      | Port 2..9                     Message data
      mask init:
      | sfcn_can_receive_mcb(canBus, outputNumber, dataType, byteOrder)
      settings: MoveFcn=drawLogos
      mask Help: web('sfcn_can_receive.html');
      mask TypeOptions canBus: CAN 1 | CAN 2
      mask TypeOptions dataType: int8 | uint8 | int16 | uint16 | int32 | uint32 | boolean
      mask Display:
      | fprintf('Receive on\nCAN %x', canBus);
      | port_label('output', 1, 'new');
      | port_label('input', 1, 'ID');patch([135 141 141],[8 14 2],[1 0 0]);patch([143 143 149],[14 2 8],[0 0 0.35]);
  Constant6 : Constant  Value=OutControl1_ID  OutDataTypeStr=uint32
  CAN_new : Outport  OutputWhenDisabled=reset  InitialOutput=0
  Out2 : Outport  Port=2  OutputWhenDisabled=reset  InitialOutput=0
  Out3 : Outport  Port=3  OutputWhenDisabled=reset  InitialOutput=0
  Out4 : Outport  Port=4  OutputWhenDisabled=reset  InitialOutput=0
  Out5 : Outport  Port=5  OutputWhenDisabled=reset  InitialOutput=0
  Out6 : Outport  Port=6  OutputWhenDisabled=reset  InitialOutput=0
  Out7 : Outport  Port=7  OutputWhenDisabled=reset  InitialOutput=0
  Out8 : Outport  Port=8  OutputWhenDisabled=reset  InitialOutput=0
  Out9 : Outport  Port=9  OutputWhenDisabled=reset  InitialOutput=0
  wires:
  CAN receive1/1(Out1) -> CAN_new/1
  CAN receive1/8(Out8) -> Out8/1
  CAN receive1/3(Out3) -> Out3/1
  CAN receive1/2(Out2) -> Out2/1
  CAN receive1/6(Out6) -> Out6/1
  CAN receive1/7(Out7) -> Out7/1
  CAN receive1/4(Out4) -> Out4/1
  CAN receive1/5(Out5) -> Out5/1
  CAN receive1/9(Out9) -> Out9/1
  Constant6/1 -> CAN receive1/1(In1)

== system HANcoder_E407_TTA_Controller_v3/HANcoder STM32 Target - E407-STM32 algorithm/Global Ticks Increment/CAN1 Recieve/RxID_CAN/OutControl2_ID_CAN ==
  Enable : EnablePort
  CAN receive1 : Subsystem  Tag=HANcoder_TARGET_STM32_E407  AncestorBlock=HANcoder_STM32_Target/STM32-E407/CAN/CAN/CAN receive  mask(CAN receive){canBus=CAN 1, outputNumber=8, dataType=uint8, byteOrder=off, tsamp=-1}
      mask prompts: canBus "CAN channel"; outputNumber "Output ports"; dataType "Output datatype"; byteOrder "Byte order: Checked = MSB first, unchecked = LSB first."; tsamp "Sample time"
      mask help:
      | Function
      | ==========
      | Receive the newest message from the specified CAN channel.
      |
      | Parameters
      | ==========
      | CAN channel:             The CAN channel to send the message on.
      | Output ports:             The amount of output ports
      | Output datatype:       The datatype of the output ports
      | Byte order:                 Select MSB or LSB first
      | Sample time:              -1 or divisible by base sample time [seconds]
      |
      | Input
      | ==========
      | Port 1:                       CAN ID(uint32) in hexadecimal ie: hex2dec('0a')
      |
      | Output
      | ==========
      | Port 1:                       Checks for new message(int8)
      | Port 2..9                     Message data
      mask init:
      | sfcn_can_receive_mcb(canBus, outputNumber, dataType, byteOrder)
      settings: MoveFcn=drawLogos
      mask Help: web('sfcn_can_receive.html');
      mask TypeOptions canBus: CAN 1 | CAN 2
      mask TypeOptions dataType: int8 | uint8 | int16 | uint16 | int32 | uint32 | boolean
      mask Display:
      | fprintf('Receive on\nCAN %x', canBus);
      | port_label('output', 1, 'new');
      | port_label('input', 1, 'ID');patch([135 141 141],[8 14 2],[1 0 0]);patch([143 143 149],[14 2 8],[0 0 0.35]);
  Constant7 : Constant  Value=OutControl2_ID  OutDataTypeStr=uint32
  CAN_new : Outport  OutputWhenDisabled=reset  InitialOutput=0
  Out2 : Outport  Port=2  OutputWhenDisabled=reset  InitialOutput=0
  Out3 : Outport  Port=3  OutputWhenDisabled=reset  InitialOutput=0
  Out4 : Outport  Port=4  OutputWhenDisabled=reset  InitialOutput=0
  Out5 : Outport  Port=5  OutputWhenDisabled=reset  InitialOutput=0
  Out6 : Outport  Port=6  OutputWhenDisabled=reset  InitialOutput=0
  Out7 : Outport  Port=7  OutputWhenDisabled=reset  InitialOutput=0
  Out8 : Outport  Port=8  OutputWhenDisabled=reset  InitialOutput=0
  Out9 : Outport  Port=9  OutputWhenDisabled=reset  InitialOutput=0
  wires:
  Constant7/1 -> CAN receive1/1(In1)
  CAN receive1/9(Out9) -> Out9/1
  CAN receive1/5(Out5) -> Out5/1
  CAN receive1/4(Out4) -> Out4/1
  CAN receive1/7(Out7) -> Out7/1
  CAN receive1/6(Out6) -> Out6/1
  CAN receive1/2(Out2) -> Out2/1
  CAN receive1/3(Out3) -> Out3/1
  CAN receive1/8(Out8) -> Out8/1
  CAN receive1/1(Out1) -> CAN_new/1

== system HANcoder_E407_TTA_Controller_v3/HANcoder STM32 Target - E407-STM32 algorithm/Global Ticks Increment/CAN1 Recieve/RxID_CAN/OutEmulator_ID_CAN ==
  Enable : EnablePort
  CAN receive1 : Subsystem  Tag=HANcoder_TARGET_STM32_E407  AncestorBlock=HANcoder_STM32_Target/STM32-E407/CAN/CAN/CAN receive  mask(CAN receive){canBus=CAN 1, outputNumber=8, dataType=uint8, byteOrder=off, tsamp=-1}
      mask prompts: canBus "CAN channel"; outputNumber "Output ports"; dataType "Output datatype"; byteOrder "Byte order: Checked = MSB first, unchecked = LSB first."; tsamp "Sample time"
      mask help:
      | Function
      | ==========
      | Receive the newest message from the specified CAN channel.
      |
      | Parameters
      | ==========
      | CAN channel:             The CAN channel to send the message on.
      | Output ports:             The amount of output ports
      | Output datatype:       The datatype of the output ports
      | Byte order:                 Select MSB or LSB first
      | Sample time:              -1 or divisible by base sample time [seconds]
      |
      | Input
      | ==========
      | Port 1:                       CAN ID(uint32) in hexadecimal ie: hex2dec('0a')
      |
      | Output
      | ==========
      | Port 1:                       Checks for new message(int8)
      | Port 2..9                     Message data
      mask init:
      | sfcn_can_receive_mcb(canBus, outputNumber, dataType, byteOrder)
      settings: MoveFcn=drawLogos
      mask Help: web('sfcn_can_receive.html');
      mask TypeOptions canBus: CAN 1 | CAN 2
      mask TypeOptions dataType: int8 | uint8 | int16 | uint16 | int32 | uint32 | boolean
      mask Display:
      | fprintf('Receive on\nCAN %x', canBus);
      | port_label('output', 1, 'new');
      | port_label('input', 1, 'ID');patch([135 141 141],[8 14 2],[1 0 0]);patch([143 143 149],[14 2 8],[0 0 0.35]);
  Constant8 : Constant  Value=OutEmulator_ID  OutDataTypeStr=uint32
  CAN_new : Outport  OutputWhenDisabled=reset  InitialOutput=0
  Out2 : Outport  Port=2  OutputWhenDisabled=reset  InitialOutput=0
  Out3 : Outport  Port=3  OutputWhenDisabled=reset  InitialOutput=0
  Out4 : Outport  Port=4  OutputWhenDisabled=reset  InitialOutput=0
  Out5 : Outport  Port=5  OutputWhenDisabled=reset  InitialOutput=0
  Out6 : Outport  Port=6  OutputWhenDisabled=reset  InitialOutput=0
  Out7 : Outport  Port=7  OutputWhenDisabled=reset  InitialOutput=0
  Out8 : Outport  Port=8  OutputWhenDisabled=reset  InitialOutput=0
  Out9 : Outport  Port=9  OutputWhenDisabled=reset  InitialOutput=0
  wires:
  CAN receive1/1(Out1) -> CAN_new/1
  CAN receive1/8(Out8) -> Out8/1
  CAN receive1/3(Out3) -> Out3/1
  CAN receive1/2(Out2) -> Out2/1
  CAN receive1/6(Out6) -> Out6/1
  CAN receive1/7(Out7) -> Out7/1
  CAN receive1/4(Out4) -> Out4/1
  CAN receive1/5(Out5) -> Out5/1
  CAN receive1/9(Out9) -> Out9/1
  Constant8/1 -> CAN receive1/1(In1)

== system HANcoder_E407_TTA_Controller_v3/HANcoder STM32 Target - E407-STM32 algorithm/Global Ticks Increment/CAN1 Recieve/RxID_CAN/SensorValues_ID_CAN ==
  Enable : EnablePort
  CAN receive1 : Subsystem  Tag=HANcoder_TARGET_STM32_E407  AncestorBlock=HANcoder_STM32_Target/STM32-E407/CAN/CAN/CAN receive  mask(CAN receive){canBus=CAN 1, outputNumber=8, dataType=uint8, byteOrder=off, tsamp=-1}
      mask prompts: canBus "CAN channel"; outputNumber "Output ports"; dataType "Output datatype"; byteOrder "Byte order: Checked = MSB first, unchecked = LSB first."; tsamp "Sample time"
      mask help:
      | Function
      | ==========
      | Receive the newest message from the specified CAN channel.
      |
      | Parameters
      | ==========
      | CAN channel:             The CAN channel to send the message on.
      | Output ports:             The amount of output ports
      | Output datatype:       The datatype of the output ports
      | Byte order:                 Select MSB or LSB first
      | Sample time:              -1 or divisible by base sample time [seconds]
      |
      | Input
      | ==========
      | Port 1:                       CAN ID(uint32) in hexadecimal ie: hex2dec('0a')
      |
      | Output
      | ==========
      | Port 1:                       Checks for new message(int8)
      | Port 2..9                     Message data
      mask init:
      | sfcn_can_receive_mcb(canBus, outputNumber, dataType, byteOrder)
      settings: MoveFcn=drawLogos
      mask Help: web('sfcn_can_receive.html');
      mask TypeOptions canBus: CAN 1 | CAN 2
      mask TypeOptions dataType: int8 | uint8 | int16 | uint16 | int32 | uint32 | boolean
      mask Display:
      | fprintf('Receive on\nCAN %x', canBus);
      | port_label('output', 1, 'new');
      | port_label('input', 1, 'ID');patch([135 141 141],[8 14 2],[1 0 0]);patch([143 143 149],[14 2 8],[0 0 0.35]);
  Constant5 : Constant  Value=SensorValues_ID  OutDataTypeStr=uint32
  CAN_new : Outport  OutputWhenDisabled=reset  InitialOutput=0
  Out2 : Outport  Port=2  OutputWhenDisabled=reset  InitialOutput=0
  Out3 : Outport  Port=3  OutputWhenDisabled=reset  InitialOutput=0
  Out4 : Outport  Port=4  OutputWhenDisabled=reset  InitialOutput=0
  Out5 : Outport  Port=5  OutputWhenDisabled=reset  InitialOutput=0
  Out6 : Outport  Port=6  OutputWhenDisabled=reset  InitialOutput=0
  Out7 : Outport  Port=7  OutputWhenDisabled=reset  InitialOutput=0
  Out8 : Outport  Port=8  OutputWhenDisabled=reset  InitialOutput=0
  Out9 : Outport  Port=9  OutputWhenDisabled=reset  InitialOutput=0
  wires:
  Constant5/1 -> CAN receive1/1(In1)
  CAN receive1/9(Out9) -> Out9/1
  CAN receive1/5(Out5) -> Out5/1
  CAN receive1/4(Out4) -> Out4/1
  CAN receive1/7(Out7) -> Out7/1
  CAN receive1/6(Out6) -> Out6/1
  CAN receive1/2(Out2) -> Out2/1
  CAN receive1/3(Out3) -> Out3/1
  CAN receive1/8(Out8) -> Out8/1
  CAN receive1/1(Out1) -> CAN_new/1

== system HANcoder_E407_TTA_Controller_v3/HANcoder STM32 Target - E407-STM32 algorithm/Global Ticks Increment/CAN1 Recieve/RxID_CAN/SetValues_ID_CAN ==
  Enable : EnablePort
  CAN receive1 : Subsystem  Tag=HANcoder_TARGET_STM32_E407  AncestorBlock=HANcoder_STM32_Target/STM32-E407/CAN/CAN/CAN receive  mask(CAN receive){canBus=CAN 1, outputNumber=8, dataType=uint8, byteOrder=off, tsamp=-1}
      mask prompts: canBus "CAN channel"; outputNumber "Output ports"; dataType "Output datatype"; byteOrder "Byte order: Checked = MSB first, unchecked = LSB first."; tsamp "Sample time"
      mask help:
      | Function
      | ==========
      | Receive the newest message from the specified CAN channel.
      |
      | Parameters
      | ==========
      | CAN channel:             The CAN channel to send the message on.
      | Output ports:             The amount of output ports
      | Output datatype:       The datatype of the output ports
      | Byte order:                 Select MSB or LSB first
      | Sample time:              -1 or divisible by base sample time [seconds]
      |
      | Input
      | ==========
      | Port 1:                       CAN ID(uint32) in hexadecimal ie: hex2dec('0a')
      |
      | Output
      | ==========
      | Port 1:                       Checks for new message(int8)
      | Port 2..9                     Message data
      mask init:
      | sfcn_can_receive_mcb(canBus, outputNumber, dataType, byteOrder)
      settings: MoveFcn=drawLogos
      mask Help: web('sfcn_can_receive.html');
      mask TypeOptions canBus: CAN 1 | CAN 2
      mask TypeOptions dataType: int8 | uint8 | int16 | uint16 | int32 | uint32 | boolean
      mask Display:
      | fprintf('Receive on\nCAN %x', canBus);
      | port_label('output', 1, 'new');
      | port_label('input', 1, 'ID');patch([135 141 141],[8 14 2],[1 0 0]);patch([143 143 149],[14 2 8],[0 0 0.35]);
  Constant4 : Constant  Value=SetValues_ID  OutDataTypeStr=uint32
  CAN_new : Outport  OutputWhenDisabled=reset  InitialOutput=0
  Out2 : Outport  Port=2  OutputWhenDisabled=reset  InitialOutput=0
  Out3 : Outport  Port=3  OutputWhenDisabled=reset  InitialOutput=0
  Out4 : Outport  Port=4  OutputWhenDisabled=reset  InitialOutput=0
  Out5 : Outport  Port=5  OutputWhenDisabled=reset  InitialOutput=0
  Out6 : Outport  Port=6  OutputWhenDisabled=reset  InitialOutput=0
  Out7 : Outport  Port=7  OutputWhenDisabled=reset  InitialOutput=0
  Out8 : Outport  Port=8  OutputWhenDisabled=reset  InitialOutput=0
  Out9 : Outport  Port=9  OutputWhenDisabled=reset  InitialOutput=0
  wires:
  CAN receive1/1(Out1) -> CAN_new/1
  CAN receive1/8(Out8) -> Out8/1
  CAN receive1/3(Out3) -> Out3/1
  CAN receive1/2(Out2) -> Out2/1
  CAN receive1/6(Out6) -> Out6/1
  CAN receive1/7(Out7) -> Out7/1
  CAN receive1/4(Out4) -> Out4/1
  CAN receive1/5(Out5) -> Out5/1
  CAN receive1/9(Out9) -> Out9/1
  Constant4/1 -> CAN receive1/1(In1)
